simulink model "Videotest"  (R2021b)
settings: Solver=VariableStepAuto  StartTime=0.0  StopTime=10  RelTol=1e-3
undefined symbols (not defined in the file): none, videoinput
libraries: visiontextngfix x1, visionstatistics x1, imaqlib x1
settings Model: Creator=rasmu  LastModifiedBy=rasmu

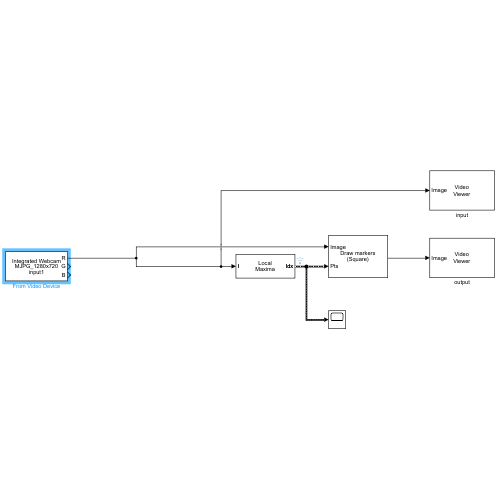
[thumbnail: Simulink's stored preview of the top-level diagram]
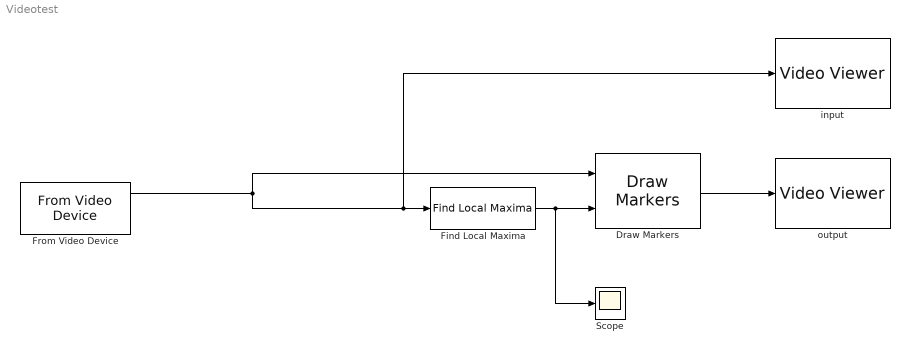
== system Videotest ==
  Draw Markers : visiontextngfix/Draw Markers  shape=Square  size=150  fill=on  fillClrSource=Specify via dialog  display=Black  intensity=200  color=[255 255 0]  opacity=0.6  viewport=Entire image  antialiasing=off  inType=Obsolete  imagePorts=One multidimensional signal  roundingMode=Floor  overflowMode=off  memoryMode=Specify word length  memoryWordLength=16  memoryFracLength=15  prodOutputMode=Binary point scaling  prodOutputWordLength=32  prodOutputFracLength=14
      settings: SourceProductBaseCode=VP
  Find Local Maxima : visionstatistics/Find Local Maxima  num_peaks=2  nhood_size=[201 201]  src_thresh=Obsolete9b  src_thresh_inuse=Specify via dialog  threshold=1  inputIsHough=off  dt_peak=uint32  isOutVarDim=on  dt_count=uint32
      settings: SourceProductBaseCode=VP
  From Video Device : imaqlib/From Video Device  DeviceMenu=winvideo 1 (Integrated Webcam)  Device=winvideo 1 (Integrated Webcam)  ObjConstructor=videoinput('winvideo', 1)  VideoFormatMenu=MJPG_1280x720  VideoFormat=MJPG_1280x720  VideoSource=input1  ROIPosition=[0 0 720 1280]  EnableHWTrigger=off  TriggerConfiguration=none/none  SampleTime=1/30  OutputPortsMode=Separate color signals  DataType=single  CanDoHWTrigger=no  ReturnedColorSpace=rgb  BlockHandle=38.0005  ROIWidth=1280  ROIHeight=720  ROIColumn=0  ROIRow=0  EngXMLPath=C:\Program Files\MATLAB\R2021b\toolbox\imaq\imaq\private  DevXMLPath=C:\ProgramData\MATLAB\SupportPackages\R2021b\toolbox\imaq\supportpackages\genericvideo\adaptor\win64  EngLibPath=C:\Program Files\MATLAB\R2021b\toolbox\imaq\imaqblks\imaqmex\win64  ColorSpace=rgb  BayerSensorAlignment=grbg  ImaqMode=off
  Scope : Scope
  input : VideoViewer  FigPos=[1 918 1536 820]
  output : VideoViewer  FigPos=[1 918 1536 820]
  wires:
  Draw Markers/1 -> output/1
  From Video Device/1 -> input/1, Find Local Maxima/1, Draw Markers/1
  Find Local Maxima/1 -> Scope/1, Draw Markers/2
